simulink model "SVPWM"  (R2020b)
settings: Solver=ode23tb  StartTime=0.0  StopTime=0.05  MaxStep=0.00001  RelTol=1e-3
libraries: simulink x1
settings Model: Creator=15070  LastModifiedBy=15070

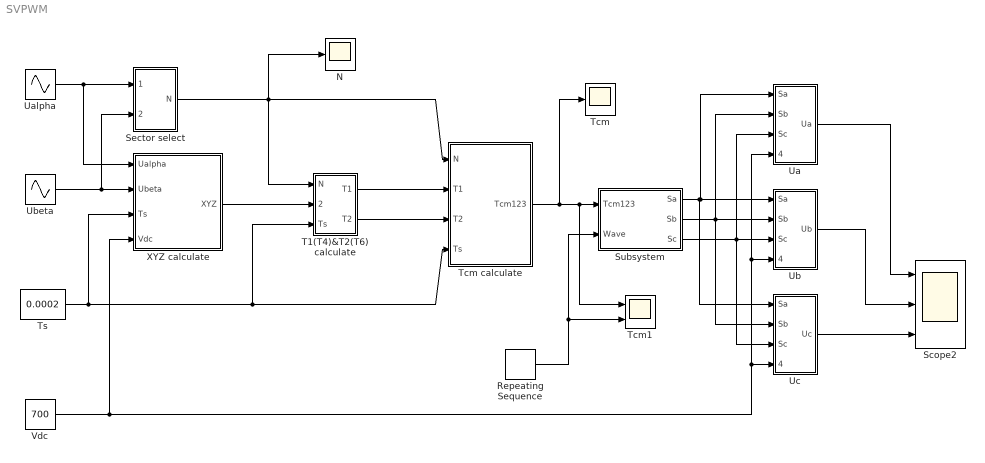
== system SVPWM ==
  N : Scope
  Repeating Sequence : simulink/Sources/Repeating Sequence  rep_seq_t=[0 1/10000 1/5000]  rep_seq_y=[0 1/10000 0]
  Scope2 : Scope  NumInputPorts=3
  Sector select : Subsystem
  Subsystem : Subsystem
  T1(T4)&T2(T6) calculate : Subsystem
  Tcm : Scope
  Tcm calculate : Subsystem
  Tcm1 : Scope  NumInputPorts=2
  Ts : Constant  Value=0.0002
  Ua : Subsystem
  Ualpha : Sin  Amplitude=200  Frequency=2*50*pi  Phase=pi/2  SampleTime=10e-6
  Ub : Subsystem
  Ubeta : Sin  Amplitude=200  Frequency=2*50*pi  SampleTime=10e-6
  Uc : Subsystem
  Vdc : Constant  Value=700
  XYZ calculate : Subsystem
  wires:
  Ubeta/1 -> XYZ calculate/2(Ubeta), Sector select/2(Ubeta)
  Ualpha/1 -> Sector select/1(Ualpha), XYZ calculate/1(Ualpha)
  Ts/1 -> T1(T4)&T2(T6) calculate/3(Ts), Tcm calculate/4(Ts), XYZ calculate/3(Ts)
  Vdc/1 -> Ua/4(Vdc), Ub/4(Vdc), Uc/4(Vdc), XYZ calculate/4(Vdc)
  XYZ calculate/1(XYZ) -> T1(T4)&T2(T6) calculate/2(XYZ)
  Sector select/1(N) -> N/1, T1(T4)&T2(T6) calculate/1(N), Tcm calculate/1(N)
  T1(T4)&T2(T6) calculate/1(T1) -> Tcm calculate/2(T1)
  T1(T4)&T2(T6) calculate/2(T2) -> Tcm calculate/3(T2)
  Tcm calculate/1(Tcm123) -> Tcm/1, Tcm1/1, Subsystem/1(Tcm123)
  Repeating Sequence/1 -> Tcm1/2, Subsystem/2(Wave)
  Subsystem/2(Sb) -> Uc/2(Sb), Ua/2(Sb), Ub/2(Sb)
  Subsystem/1(Sa) -> Uc/1(Sa), Ua/1(Sa), Ub/1(Sa)
  Subsystem/3(Sc) -> Uc/3(Sc), Ua/3(Sc), Ub/3(Sc)
  Ua/1(Ua) -> Scope2/1
  Ub/1(Ub) -> Scope2/2
  Uc/1(Uc) -> Scope2/3

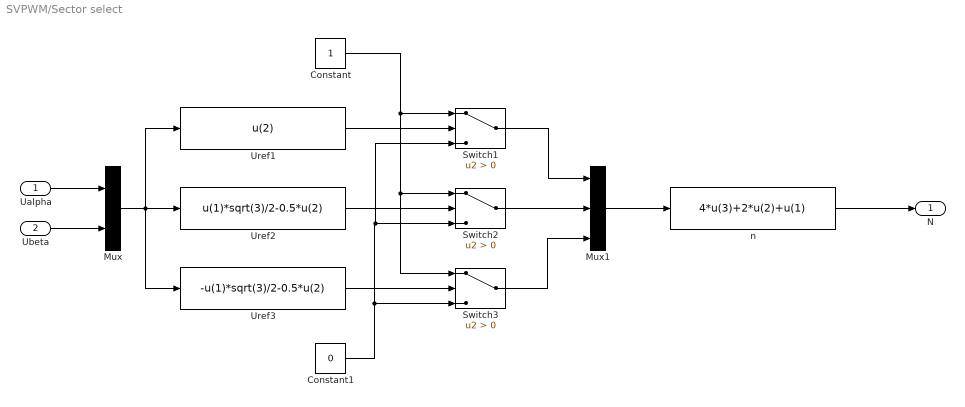
== system SVPWM/Sector select ==
  Ualpha : Inport
  Ubeta : Inport  Port=2
  Constant : Constant
  Constant1 : Constant  Value=0
  Mux : Mux  Inputs=2
  Mux1 : Mux  Inputs=3
  Switch1 : Switch  Criteria=u2 > Threshold
  Switch2 : Switch  Criteria=u2 > Threshold
  Switch3 : Switch  Criteria=u2 > Threshold
  Uref1 : Fcn  Expr=u(2)
  Uref2 : Fcn  Expr=u(1)*sqrt(3)/2-0.5*u(2)
  Uref3 : Fcn  Expr=-u(1)*sqrt(3)/2-0.5*u(2)
  n : Fcn  Expr=4*u(3)+2*u(2)+u(1)
  N : Outport
  wires:
  Switch3/1 -> Mux1/3
  Mux/1 -> Uref1/1, Uref3/1, Uref2/1
  Ualpha/1 -> Mux/1
  Uref1/1 -> Switch1/2
  Ubeta/1 -> Mux/2
  Constant/1 -> Switch3/1, Switch2/1, Switch1/1
  Switch1/1 -> Mux1/1
  Mux1/1 -> n/1
  Constant1/1 -> Switch3/3, Switch1/3, Switch2/3
  Uref3/1 -> Switch3/2
  n/1 -> N/1
  Switch2/1 -> Mux1/2
  Uref2/1 -> Switch2/2

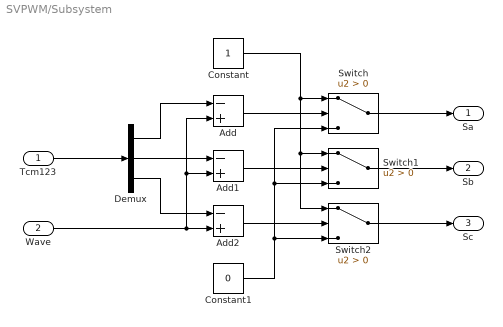
== system SVPWM/Subsystem ==
  Tcm123 : Inport
  Wave : Inport  Port=2
  Add : Sum  Inputs=-+
  Add1 : Sum  Inputs=-+
  Add2 : Sum  Inputs=-+
  Constant : Constant
  Constant1 : Constant  Value=0
  Demux : Demux  Outputs=3
  Switch : Switch  Criteria=u2 > Threshold
  Switch1 : Switch  Criteria=u2 > Threshold
  Switch2 : Switch  Criteria=u2 > Threshold
  Sa : Outport
  Sb : Outport  Port=2
  Sc : Outport  Port=3
  wires:
  Constant1/1 -> Switch2/3, Switch/3, Switch1/3
  Wave/1 -> Add1/2, Add/2, Add2/2
  Constant/1 -> Switch1/1, Switch2/1, Switch/1
  Add2/1 -> Switch2/2
  Add1/1 -> Switch1/2
  Tcm123/1 -> Demux/1
  Switch2/1 -> Sc/1
  Switch/1 -> Sa/1
  Add/1 -> Switch/2
  Switch1/1 -> Sb/1
  Demux/2 -> Add1/1
  Demux/3 -> Add2/1
  Demux/1 -> Add/1

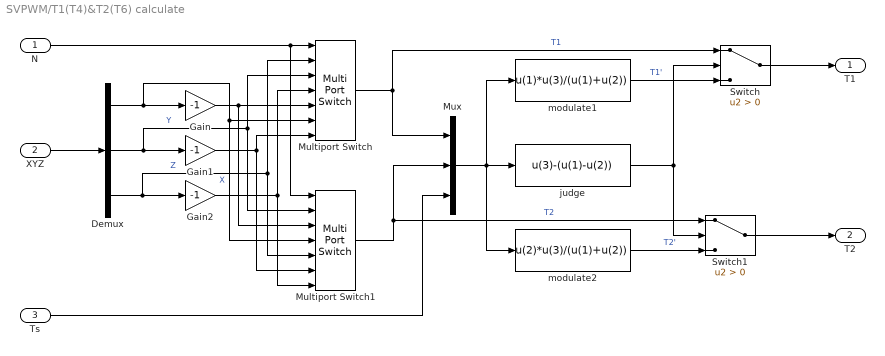
== system SVPWM/T1(T4)&T2(T6) calculate ==
  N : Inport
  XYZ : Inport  Port=2
  Ts : Inport  Port=3
  Demux : Demux  Outputs=3
  Gain : Gain  Gain=-1
  Gain1 : Gain  Gain=-1
  Gain2 : Gain  Gain=-1
  Multiport Switch : MultiPortSwitch  Inputs=6
  Multiport Switch1 : MultiPortSwitch  Inputs=6
  Mux : Mux  Inputs=3
  Switch : Switch  Criteria=u2 > Threshold
  Switch1 : Switch  Criteria=u2 > Threshold
  judge : Fcn  Expr=u(3)-(u(1)-u(2))
  modulate1 : Fcn  Expr=u(1)*u(3)/(u(1)+u(2))
  modulate2 : Fcn  Expr=u(2)*u(3)/(u(1)+u(2))
  T1 : Outport
  T2 : Outport  Port=2
  wires:
  XYZ/1 -> Demux/1
  Mux/1 -> modulate2/1, judge/1, modulate1/1
  Multiport Switch/1 -> Mux/1, Switch/1  "T1"
  Gain/1 -> Multiport Switch/5, Multiport Switch1/3
  judge/1 -> Switch/2, Switch1/2
  Demux/3 -> Gain2/1, Multiport Switch/2, Multiport Switch1/5  "Z"
  N/1 -> Multiport Switch1/1, Multiport Switch/1
  Demux/1 -> Gain/1, Multiport Switch/6, Multiport Switch1/4  "X"
  Gain1/1 -> Multiport Switch/7, Multiport Switch1/6
  Gain2/1 -> Multiport Switch/4, Multiport Switch1/7
  Ts/1 -> Mux/3
  modulate2/1 -> Switch1/3  "T2'"
  modulate1/1 -> Switch/3  "T1'"
  Demux/2 -> Multiport Switch/3, Multiport Switch1/2, Gain1/1  "Y"
  Switch/1 -> T1/1
  Multiport Switch1/1 -> Mux/2, Switch1/1  "T2"
  Switch1/1 -> T2/1

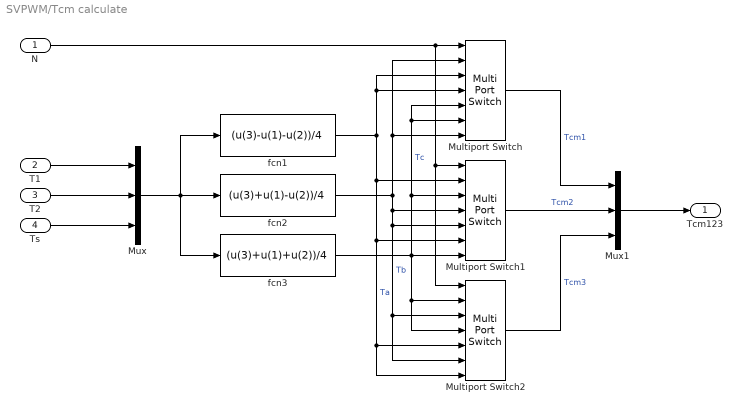
== system SVPWM/Tcm calculate ==
  N : Inport
  T1 : Inport  Port=2
  T2 : Inport  Port=3
  Ts : Inport  Port=4
  Multiport Switch : MultiPortSwitch  Inputs=6
  Multiport Switch1 : MultiPortSwitch  Inputs=6
  Multiport Switch2 : MultiPortSwitch  Inputs=6
  Mux : Mux  Inputs=3
  Mux1 : Mux  Inputs=3
  fcn1 : Fcn  Expr=(u(3)-u(1)-u(2))/4
  fcn2 : Fcn  Expr=(u(3)+u(1)-u(2))/4
  fcn3 : Fcn  Expr=(u(3)+u(1)+u(2))/4
  Tcm123 : Outport
  wires:
  fcn1/1 -> Multiport Switch2/7, Multiport Switch2/5, Multiport Switch1/6, Multiport Switch1/2, Multiport Switch/4, Multiport Switch/3  "Ta"
  Mux/1 -> fcn2/1, fcn1/1, fcn3/1
  fcn2/1 -> Multiport Switch2/6, Multiport Switch2/3, Multiport Switch1/5, Multiport Switch1/4, Multiport Switch/7, Multiport Switch/2  "Tb"
  N/1 -> Multiport Switch2/1, Multiport Switch1/1, Multiport Switch/1
  fcn3/1 -> Multiport Switch2/4, Multiport Switch2/2, Multiport Switch1/7, Multiport Switch/5, Multiport Switch/6, Multiport Switch1/3  "Tc"
  Mux1/1 -> Tcm123/1
  T1/1 -> Mux/1
  Multiport Switch/1 -> Mux1/1  "Tcm1"
  T2/1 -> Mux/2
  Ts/1 -> Mux/3
  Multiport Switch1/1 -> Mux1/2  "Tcm2"
  Multiport Switch2/1 -> Mux1/3  "Tcm3"

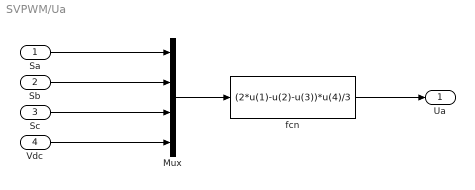
== system SVPWM/Ua ==
  Sa : Inport
  Sb : Inport  Port=2
  Sc : Inport  Port=3
  Vdc : Inport  Port=4
  Mux : Mux
  fcn : Fcn  Expr=(2*u(1)-u(2)-u(3))*u(4)/3
  Ua : Outport
  wires:
  Sb/1 -> Mux/2
  Mux/1 -> fcn/1
  Vdc/1 -> Mux/4
  Sc/1 -> Mux/3
  Sa/1 -> Mux/1
  fcn/1 -> Ua/1

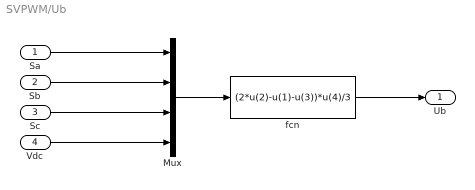
== system SVPWM/Ub ==
  Sa : Inport
  Sb : Inport  Port=2
  Sc : Inport  Port=3
  Vdc : Inport  Port=4
  Mux : Mux
  fcn : Fcn  Expr=(2*u(2)-u(1)-u(3))*u(4)/3
  Ub : Outport
  wires:
  Sb/1 -> Mux/2
  Mux/1 -> fcn/1
  Vdc/1 -> Mux/4
  Sc/1 -> Mux/3
  Sa/1 -> Mux/1
  fcn/1 -> Ub/1

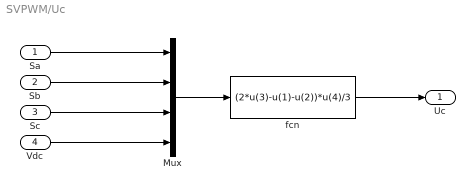
== system SVPWM/Uc ==
  Sa : Inport
  Sb : Inport  Port=2
  Sc : Inport  Port=3
  Vdc : Inport  Port=4
  Mux : Mux
  fcn : Fcn  Expr=(2*u(3)-u(1)-u(2))*u(4)/3
  Uc : Outport
  wires:
  Sb/1 -> Mux/2
  Mux/1 -> fcn/1
  Vdc/1 -> Mux/4
  Sc/1 -> Mux/3
  Sa/1 -> Mux/1
  fcn/1 -> Uc/1

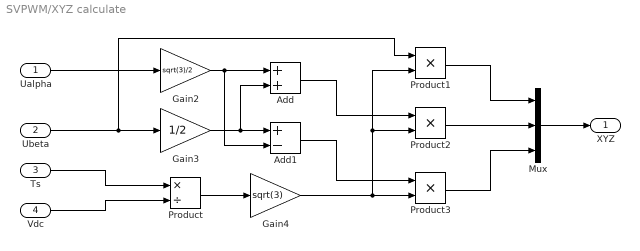
== system SVPWM/XYZ calculate ==
  Ualpha : Inport
  Ubeta : Inport  Port=2
  Ts : Inport  Port=3
  Vdc : Inport  Port=4
  Add : Sum
  Add1 : Sum  Inputs=+-
  Gain2 : Gain  Gain=sqrt(3)/2
  Gain3 : Gain  Gain=1/2
  Gain4 : Gain  Gain=sqrt(3)
  Mux : Mux  Inputs=3
  Product : Product  Inputs=*/
  Product1 : Product  Inputs=**
  Product2 : Product  Inputs=**
  Product3 : Product  Inputs=**
  XYZ : Outport
  wires:
  Ts/1 -> Product/1
  Ualpha/1 -> Gain2/1
  Add1/1 -> Product3/1
  Gain3/1 -> Add1/1, Add/2
  Add/1 -> Product2/1
  Gain4/1 -> Product1/2, Product2/2, Product3/2
  Gain2/1 -> Add1/2, Add/1
  Ubeta/1 -> Product1/1, Gain3/1
  Product3/1 -> Mux/3
  Vdc/1 -> Product/2
  Product1/1 -> Mux/1
  Product2/1 -> Mux/2
  Product/1 -> Gain4/1
  Mux/1 -> XYZ/1
